simulink model "HW7_F_f_a"  (R2018a)
settings: Solver=VariableStepAuto  StartTime=0.0  StopTime=100  RelTol=1e-3
InitFcn:
  | vtol_param
  | F_f
StartFcn:
  | vtol_param
  | F_f
undefined symbols (not defined in the file or in its folder): Kh, P, phlead, PlotVtol, zhlead
settings Model: Creator=sadam  LastModifiedBy=sadam

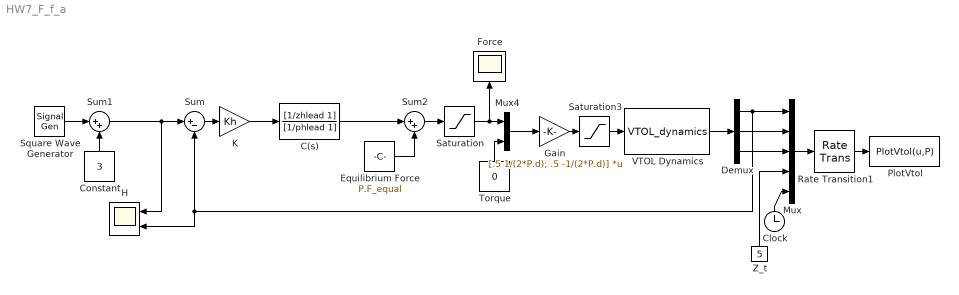
== system HW7_F_f_a ==
  C(s) : TransferFcn  Numerator=[1/zhlead 1]  Denominator=[1/phlead 1]
  Clock : Clock
  Constant : Constant  Value=3
  Demux : Demux  Outputs=3
  Equilibrium Force : Constant  Value=P.F_equal
  "Force " : Scope
  Gain : Gain  Gain=[.5 1/(2*P.d); .5 -1/(2*P.d)]  Multiplication=Matrix(K*u)
  "H " : Scope  NumInputPorts=2
  K : Gain  Gain=Kh
  Mux : Mux  Inputs=5
  Mux4 : Mux  Inputs=2
  "PlotVtol " : MATLABFcn  MATLABFcn=PlotVtol(u,P)  OutputDimensions=0
  Rate Transition1 : RateTransition  OutPortSampleTime=P.t_plot
  Saturation : Saturate  UpperLimit=P.Force_max  LowerLimit=-P.Force_max
  Saturation3 : Saturate  UpperLimit=P.Force_max  LowerLimit=-P.Force_max
  Square Wave Generator : SignalGenerator  WaveForm=square  Amplitude=2.5  Frequency=0.05
  Sum : Sum  Inputs=|+-
  Sum1 : Sum  Inputs=|++
  Sum2 : Sum  Inputs=|++
  Torque : Constant  Value=0
  VTOL Dynamics : S-Function  FunctionName=VTOL_dynamics  Parameters=P  SFunctionDeploymentMode=off  EnableBusSupport=off
  Z_t : Constant  Value=5
  wires:
  Demux/2 -> Mux/2
  Demux/3 -> Mux/3
  Demux/1 -> "H "/2, Sum/2, Mux/1
  Saturation3/1 -> VTOL Dynamics/1
  Rate Transition1/1 -> "PlotVtol "/1
  Mux/1 -> Rate Transition1/1
  Clock/1 -> Mux/5
  Z_t/1 -> Mux/4
  VTOL Dynamics/1 -> Demux/1
  Mux4/1 -> Gain/1
  Gain/1 -> Saturation3/1
  K/1 -> C(s)/1
  Torque/1 -> Mux4/2
  Sum/1 -> K/1
  Equilibrium Force/1 -> Sum2/2
  Sum2/1 -> Saturation/1
  Saturation/1 -> "Force "/1, Mux4/1
  C(s)/1 -> Sum2/1
  Square Wave Generator/1 -> Sum1/1
  Sum1/1 -> "H "/1, Sum/1
  Constant/1 -> Sum1/2
